simulink model "subsystem_118_bus"  (R2025b)
settings: Solver=ode45  StartTime=0.0  StopTime=Tstop  FixedStep=Ts  RelTol=1e-12  AbsTol=1e-12
values from neighbouring files (symbols this model uses):
  Imax = 15    [config_file.m]
  nominalInter =     [nominalInter.mat]
  nominalU =     [nominalU.mat]
  nominalY =     [nominalY.mat]
  sub = struct    [main_sub_118_bus.m]
  sys_j = sys_j(1:end-1)    [IBR_modelGenerator.m]
  sys_j_AA = sys_j    [modularMOR_main.m]
  sys_j_BT = sys_j    [modularMOR_main.m]
  Tstep_gfl = 0.1    [main_sub_118_bus.m]
  Tstep_gfm = 0.1    [main_sub_118_bus.m]
  w = 2*pi*50    (= 314.159265359)    [config_file.m]    (also in mirrorMimoWeightedFrequencyData.m = w(:); modularMOR_main.m = w(:).'; plotTest.m = w(:).')
undefined symbols (not defined in the file or in its folder): con_sub, linSys1, linSys2, linSys3
libraries: simulink x10
(part 6 of 6)

== system subsystem_118_bus/Subsystem3/area3/ibr/gfl/pll_pi ==
  "  " : Inport
  Integrator : Integrator  ContinuousStateAttributes='gfl_pll'
  Ki : Gain  Gain=Subsystem.gfl_gains.kipll
  Kp : Gain  Gain=Subsystem.gfl_gains.kppll
  Sum : Sum  Inputs=|++
  " " : Outport
  wires:
  Kp/1 -> Sum/1
  Integrator/1 -> Sum/2
  Ki/1 -> Integrator/1
  "  "/1 -> Ki/1, Kp/1
  Sum/1 -> " "/1

== system subsystem_118_bus/Subsystem3/area3/ibr/gfl/simplified current loop d-axis ==
  " " : Inport
  Gain : Gain  Gain=Subsystem.gfl.i_loop_w
  Integrator1 : Integrator  InitialCondition=Subsystem.gfl.i_d  ContinuousStateAttributes='gfl_id_ctrl'
  Sum2 : Sum  Inputs=-+
  "  " : Outport
  wires:
  Gain/1 -> Integrator1/1
  Integrator1/1 -> "  "/1, Sum2/1
  Sum2/1 -> Gain/1
  " "/1 -> Sum2/2

== system subsystem_118_bus/Subsystem3/area3/ibr/gfl/simplified current loop q-axis ==
  i_gfl_q : Inport
  Gain : Gain  Gain=Subsystem.gfl.i_loop_w
  Integrator1 : Integrator  InitialCondition=Subsystem.gfl.i_q  ContinuousStateAttributes='gfl_iq_ctrl'
  Sum2 : Sum  Inputs=-+
  igfl_q : Outport
  wires:
  Gain/1 -> Integrator1/1
  Integrator1/1 -> igfl_q/1, Sum2/1
  Sum2/1 -> Gain/1
  i_gfl_q/1 -> Sum2/2

== system subsystem_118_bus/Subsystem3/area3/ibr/gfl/v measurement delay ==
  in : Inport
  Integrator1 : Integrator  InitialCondition=Subsystem.gfl.v_ref  ContinuousStateAttributes='gfl_v_m'
  Sum2 : Sum  Inputs=-+
  v_meas_bw : Gain  Gain=Subsystem.gfl.v_meas_w
  out : Outport
  wires:
  in/1 -> Sum2/2
  Sum2/1 -> v_meas_bw/1
  Integrator1/1 -> Sum2/1, out/1
  v_meas_bw/1 -> Integrator1/1

== system subsystem_118_bus/Subsystem3/area3/ibr/gfl/v_loop_pi ==
  "  " : Inport
  Integrator : Integrator  ContinuousStateAttributes='gfl_v_ctrl'
  Ki : Gain  Gain=Subsystem.gfl_gains.kiv
  Kp : Gain  Gain=Subsystem.gfl_gains.kpv
  Sum : Sum  Inputs=|++
  " " : Outport
  wires:
  Kp/1 -> Sum/1
  Integrator/1 -> Sum/2
  Ki/1 -> Integrator/1
  "  "/1 -> Ki/1, Kp/1
  Sum/1 -> " "/1

== system subsystem_118_bus/Subsystem3/area3/ibr/gfm/DQ//dq ==
  D_quantity : Inport
  Q_quantity : Inport  Port=2
  theta : Inport  Port=3
  Complex to Magnitude-Angle : ComplexToMagnitudeAngle
  Complex to Real-Imag : ComplexToRealImag
  Magnitude-Angle to Complex : MagnitudeAngleToComplex
  Real-Imag to Complex : RealImagToComplex
  Sum : Sum  Inputs=|+-
  d_quantity : Outport
  q_quantity : Outport  Port=2
  wires:
  D_quantity/1 -> Real-Imag to Complex/1
  Complex to Magnitude-Angle/2 -> Sum/1
  Complex to Magnitude-Angle/1 -> Magnitude-Angle to Complex/1
  Real-Imag to Complex/1 -> Complex to Magnitude-Angle/1
  Sum/1 -> Magnitude-Angle to Complex/2
  Q_quantity/1 -> Real-Imag to Complex/2
  Magnitude-Angle to Complex/1 -> Complex to Real-Imag/1
  Complex to Real-Imag/1 -> d_quantity/1
  Complex to Real-Imag/2 -> q_quantity/1
  theta/1 -> Sum/2

== system subsystem_118_bus/Subsystem3/area3/ibr/gfm/Subsystem1 ==
  vbDQ : Inport
  IbDQ : Inport  Port=2
  Complex to Real-Imag : ComplexToRealImag
  Complex to Real-Imag1 : ComplexToRealImag
  Product{,1..3} (4 alike) : Product
  Sum : Sum
  Sum1 : Sum  Inputs=+-
  Pm : Outport
  Qm : Outport  Port=2
  wires:
  Product/1 -> Sum/1
  Product1/1 -> Sum/2
  Sum/1 -> Pm/1
  Sum1/1 -> Qm/1
  Product3/1 -> Sum1/2
  Product2/1 -> Sum1/1
  [vbQ] -> Product2/1
  [IbD] -> Product2/2
  [vbD] -> Product3/1
  [IbQ] -> Product3/2
  [vbD] -> Product/1
  [IbD] -> Product/2
  [IbQ] -> Product1/2
  [vbQ] -> Product1/1
  vbDQ/1 -> Complex to Real-Imag/1
  Complex to Real-Imag/1 -> [vbD]
  Complex to Real-Imag/2 -> [vbQ]
  IbDQ/1 -> Complex to Real-Imag1/1
  Complex to Real-Imag1/1 -> [IbD]
  Complex to Real-Imag1/2 -> [IbQ]

== system subsystem_118_bus/Subsystem3/area3/ibr/gfm/dq//DQ ==
  d-quantity : Inport
  q-quantity : Inport  Port=2
  theta : Inport  Port=3
  Complex to Magnitude-Angle : ComplexToMagnitudeAngle
  Complex to Real-Imag : ComplexToRealImag
  Magnitude-Angle to Complex : MagnitudeAngleToComplex
  Real-Imag to Complex : RealImagToComplex
  Sum : Sum  Inputs=|++
  D-quantity : Outport
  Q-quantity : Outport  Port=2
  wires:
  d-quantity/1 -> Real-Imag to Complex/1
  Complex to Magnitude-Angle/2 -> Sum/1
  Complex to Magnitude-Angle/1 -> Magnitude-Angle to Complex/1
  Real-Imag to Complex/1 -> Complex to Magnitude-Angle/1
  Sum/1 -> Magnitude-Angle to Complex/2
  q-quantity/1 -> Real-Imag to Complex/2
  Magnitude-Angle to Complex/1 -> Complex to Real-Imag/1
  Complex to Real-Imag/1 -> D-quantity/1
  Complex to Real-Imag/2 -> Q-quantity/1
  theta/1 -> Sum/2

== system subsystem_118_bus/Subsystem3/area3/ibr/gfm/filter capacitor dynamics ==
  i_cf_d : Inport
  w : Inport  Port=2
  i_cf_q : Inport  Port=3
  1/C_gfm : Gain  Gain=1./Subsystem.gfm.c
  "1/C_gfm " : Gain  Gain=1./Subsystem.gfm.c
  Display : Display
  Integrator : Integrator  InitialCondition=Subsystem.gfm.v_d  ContinuousStateAttributes='gfm_vd'
  Integrator1 : Integrator  InitialCondition=Subsystem.gfm.v_q  ContinuousStateAttributes='gfm_vq'
  Product : Product
  Product1 : Product
  Sum2 : Sum  Inputs=+-
  Sum3 : Sum
  v_gfl_d : Outport
  v_gfl_q : Outport  Port=2
  wires:
  w/1 -> [ws]
  [ws] -> Product/1
  Integrator/1 -> Product1/1, v_gfl_d/1
  Integrator1/1 -> Product/2, v_gfl_q/1
  [ws] -> Product1/2
  Sum3/1 -> Display/1, Integrator/1
  Sum2/1 -> Integrator1/1
  1/C_gfm/1 -> Sum3/2
  Product/1 -> Sum3/1
  "1/C_gfm "/1 -> Sum2/1
  Product1/1 -> Sum2/2
  i_cf_d/1 -> 1/C_gfm/1
  i_cf_q/1 -> "1/C_gfm "/1

== system subsystem_118_bus/Subsystem3/area3/ibr/gfm/p measurement delay ==
  in : Inport
  Integrator1 : Integrator  InitialCondition=Subsystem.gfm.p_ref  ContinuousStateAttributes='gfm_p_m'
  Sum2 : Sum  Inputs=-+
  p_meas_bw : Gain  Gain=Subsystem.gfm.p_meas_w
  out : Outport
  wires:
  in/1 -> Sum2/2
  Sum2/1 -> p_meas_bw/1
  Integrator1/1 -> Sum2/1, out/1
  p_meas_bw/1 -> Integrator1/1

== system subsystem_118_bus/Subsystem3/area3/ibr/gfm/q measurement delay ==
  in : Inport
  Integrator1 : Integrator  InitialCondition=Subsystem.gfm.q_ref  ContinuousStateAttributes='gfm_q_m'
  Sum2 : Sum  Inputs=-+
  p_meas_bw : Gain  Gain=Subsystem.gfm.p_meas_w
  out : Outport
  wires:
  p_meas_bw/1 -> Integrator1/1
  Integrator1/1 -> out/1, Sum2/1
  Sum2/1 -> p_meas_bw/1
  in/1 -> Sum2/2

== system subsystem_118_bus/Subsystem3/area3/ibr/gfm/simplified current loop d-axis ==
  " " : Inport
  Display : Display
  Gain : Gain  Gain=Subsystem.gfm.i_loop_w
  Integrator1 : Integrator  InitialCondition=Subsystem.gfm.i_d  ContinuousStateAttributes='gfm_id_ctrl'
  Sum2 : Sum  Inputs=-+
  "  " : Outport
  wires:
  Gain/1 -> Display/1, Integrator1/1
  Integrator1/1 -> "  "/1, Sum2/1
  Sum2/1 -> Gain/1
  " "/1 -> Sum2/2

== system subsystem_118_bus/Subsystem3/area3/ibr/gfm/simplified current loop q-axis ==
  " " : Inport
  Gain : Gain  Gain=Subsystem.gfm.i_loop_w
  Integrator1 : Integrator  InitialCondition=Subsystem.gfm.i_q  ContinuousStateAttributes='gfm_iq_ctrl'
  Sum2 : Sum  Inputs=-+
  "  " : Outport
  wires:
  " "/1 -> Sum2/2
  Sum2/1 -> Gain/1
  Integrator1/1 -> Sum2/1, "  "/1
  Gain/1 -> Integrator1/1

== system subsystem_118_bus/Subsystem3/area3/ibr/gfm/v measurement delay ==
  in : Inport
  Integrator1 : Integrator  InitialCondition=Subsystem.gfm.v_ref  ContinuousStateAttributes='gfm_v_m'
  Sum2 : Sum  Inputs=-+
  v_meas_bw : Gain  Gain=Subsystem.gfm.q_meas_w
  out : Outport
  wires:
  v_meas_bw/1 -> Integrator1/1
  Integrator1/1 -> out/1, Sum2/1
  Sum2/1 -> v_meas_bw/1
  in/1 -> Sum2/2

== system subsystem_118_bus/Subsystem3/area3/ibr/gfm/vd_loop_pi ==
  "  " : Inport
  Integrator : Integrator  ContinuousStateAttributes='gfm_vd_ctrl'
  Ki : Gain  Gain=Subsystem.gfm_gains.vd_ki
  Kp : Gain  Gain=Subsystem.gfm_gains.vd_kp
  Sum : Sum  Inputs=|++
  " " : Outport
  wires:
  Kp/1 -> Sum/1
  Integrator/1 -> Sum/2
  Ki/1 -> Integrator/1
  "  "/1 -> Ki/1, Kp/1
  Sum/1 -> " "/1

== system subsystem_118_bus/Subsystem3/area3/ibr/gfm/vq_loop_pi ==
  "  " : Inport
  Integrator : Integrator  ContinuousStateAttributes='gfm_vq_ctrl'
  Ki : Gain  Gain=Subsystem.gfm_gains.vq_ki
  Kp : Gain  Gain=Subsystem.gfm_gains.vq_kp
  Sum : Sum  Inputs=|++
  " " : Outport
  wires:
  Sum/1 -> " "/1
  "  "/1 -> Kp/1, Ki/1
  Ki/1 -> Integrator/1
  Integrator/1 -> Sum/2
  Kp/1 -> Sum/1

== system subsystem_118_bus/Subsystem3/area3/non_ibr/floating buses/line charging dynamics ==
  note: I am multiplying here by negative
  note: I am multiplying here by negative
  i_float_D : Inport
  i_float_Q : Inport  Port=2
  " " : Integrator  InitialCondition=Subsystem.float.v_D  ContinuousStateAttributes='floatvD'
  1/C_float : Gain  Gain=-1./Subsystem.float.c
  "1/C_float " : Gain  Gain=-1./Subsystem.float.c
  Constant : Constant  Value=w
  Integrator1 : Integrator  InitialCondition=Subsystem.float.v_Q  ContinuousStateAttributes='floatvQ'
  Product : Product
  Product1 : Product
  Sum2 : Sum  Inputs=+-
  Sum3 : Sum
  v_float_D : Outport
  v_float_Q : Outport  Port=2
  wires:
  " "/1 -> Product1/1, v_float_D/1
  Integrator1/1 -> v_float_Q/1, Product/2
  [ws] -> Product1/2
  Sum3/1 -> " "/1
  Sum2/1 -> Integrator1/1
  1/C_float/1 -> Sum3/2
  Product/1 -> Sum3/1
  "1/C_float "/1 -> Sum2/1
  Product1/1 -> Sum2/2
  i_float_D/1 -> 1/C_float/1
  i_float_Q/1 -> "1/C_float "/1
  [ws] -> Product/1
  Constant/1 -> [ws]

== system subsystem_118_bus/Subsystem3/area3/non_ibr/load buses/Subsystem ==
  p : Inport
  q : Inport  Port=2
  vD : Inport  Port=3
  vQ : Inport  Port=4
  Complex to Real-Imag : ComplexToRealImag
  Conj : Math  Operator=conj
  Divide : Product  Inputs=*/
  Real-Imag to Complex : RealImagToComplex
  Real-Imag to Complex1 : RealImagToComplex
  i_inj_load_d : Outport
  i_inj_load_q : Outport  Port=2
  wires:
  q/1 -> Real-Imag to Complex/2
  Real-Imag to Complex1/1 -> Divide/2
  Divide/1 -> Conj/1
  Complex to Real-Imag/2 -> i_inj_load_q/1
  Real-Imag to Complex/1 -> Divide/1
  vQ/1 -> Real-Imag to Complex1/2
  vD/1 -> Real-Imag to Complex1/1
  Complex to Real-Imag/1 -> i_inj_load_d/1
  p/1 -> Real-Imag to Complex/1
  Conj/1 -> Complex to Real-Imag/1

== system subsystem_118_bus/Subsystem3/area3/non_ibr/load buses/line charging dynamics ==
  i_load_c_D : Inport
  i_load_c_Q : Inport  Port=2
  " " : Integrator  InitialCondition=Subsystem.load1.v_D  ContinuousStateAttributes='loadvD'
  1/C_load : Gain  Gain=1./Subsystem.load1.c
  "1/C_load " : Gain  Gain=1./Subsystem.load1.c
  Constant : Constant  Value=w
  Integrator1 : Integrator  InitialCondition=Subsystem.load1.v_Q  ContinuousStateAttributes='loadvQ'
  Product : Product
  Product1 : Product
  Sum2 : Sum  Inputs=+-
  Sum3 : Sum
  v_load_D : Outport
  v_load_Q : Outport  Port=2
  wires:
  [ws] -> Product/1
  " "/1 -> Product1/1, v_load_D/1
  Integrator1/1 -> v_load_Q/1, Product/2
  [ws] -> Product1/2
  Sum3/1 -> " "/1
  Sum2/1 -> Integrator1/1
  1/C_load/1 -> Sum3/2
  Product/1 -> Sum3/1
  "1/C_load "/1 -> Sum2/1
  Product1/1 -> Sum2/2
  i_load_c_D/1 -> 1/C_load/1
  i_load_c_Q/1 -> "1/C_load "/1
  Constant/1 -> [ws]

== system subsystem_118_bus/Linear 118 Bus FOM/Subsystem3/area3/ibr/gfl/DQ//dq ==
  D_quantity : Inport
  Q_quantity : Inport  Port=2
  theta : Inport  Port=3
  Complex to Magnitude-Angle : ComplexToMagnitudeAngle
  Complex to Real-Imag : ComplexToRealImag
  Magnitude-Angle to Complex : MagnitudeAngleToComplex
  Real-Imag to Complex : RealImagToComplex
  Sum : Sum  Inputs=|+-
  d_quantity : Outport
  q_quantity : Outport  Port=2
  wires:
  D_quantity/1 -> Real-Imag to Complex/1
  Complex to Magnitude-Angle/2 -> Sum/1
  Complex to Magnitude-Angle/1 -> Magnitude-Angle to Complex/1
  Real-Imag to Complex/1 -> Complex to Magnitude-Angle/1
  Sum/1 -> Magnitude-Angle to Complex/2
  Q_quantity/1 -> Real-Imag to Complex/2
  Magnitude-Angle to Complex/1 -> Complex to Real-Imag/1
  Complex to Real-Imag/1 -> d_quantity/1
  Complex to Real-Imag/2 -> q_quantity/1
  theta/1 -> Sum/2

== system subsystem_118_bus/Linear 118 Bus FOM/Subsystem3/area3/ibr/gfl/Subsystem ==
  vbDQ : Inport
  Abs : Abs  SaturateOnIntegerOverflow=off
  Vm : Outport
  wires:
  Abs/1 -> Vm/1
  vbDQ/1 -> Abs/1

== system subsystem_118_bus/Linear 118 Bus FOM/Subsystem3/area3/ibr/gfl/Subsystem1 ==
  vbDQ : Inport
  IbDQ : Inport  Port=2
  Complex to Real-Imag : ComplexToRealImag
  Complex to Real-Imag1 : ComplexToRealImag
  Product{,1..3} (4 alike) : Product
  Sum : Sum
  Sum1 : Sum  Inputs=+-
  Pm : Outport
  Qm : Outport  Port=2
  wires:
  Product/1 -> Sum/1
  Product1/1 -> Sum/2
  Sum/1 -> Pm/1
  Sum1/1 -> Qm/1
  Product3/1 -> Sum1/2
  Product2/1 -> Sum1/1
  [vbQ] -> Product2/1
  [IbD] -> Product2/2
  [vbD] -> Product3/1
  [IbQ] -> Product3/2
  [vbD] -> Product/1
  [IbD] -> Product/2
  [IbQ] -> Product1/2
  [vbQ] -> Product1/1
  vbDQ/1 -> Complex to Real-Imag/1
  Complex to Real-Imag/1 -> [vbD]
  Complex to Real-Imag/2 -> [vbQ]
  IbDQ/1 -> Complex to Real-Imag1/1
  Complex to Real-Imag1/1 -> [IbD]
  Complex to Real-Imag1/2 -> [IbQ]

== system subsystem_118_bus/Linear 118 Bus FOM/Subsystem3/area3/ibr/gfl/dq//DQ ==
  d-quantity : Inport
  q-quantity : Inport  Port=2
  theta : Inport  Port=3
  Complex to Magnitude-Angle : ComplexToMagnitudeAngle
  Complex to Real-Imag : ComplexToRealImag
  Magnitude-Angle to Complex : MagnitudeAngleToComplex
  Real-Imag to Complex : RealImagToComplex
  Sum : Sum  Inputs=|++
  D-quantity : Outport
  Q-quantity : Outport  Port=2
  wires:
  d-quantity/1 -> Real-Imag to Complex/1
  Complex to Magnitude-Angle/2 -> Sum/1
  Complex to Magnitude-Angle/1 -> Magnitude-Angle to Complex/1
  Real-Imag to Complex/1 -> Complex to Magnitude-Angle/1
  Sum/1 -> Magnitude-Angle to Complex/2
  q-quantity/1 -> Real-Imag to Complex/2
  Magnitude-Angle to Complex/1 -> Complex to Real-Imag/1
  Complex to Real-Imag/1 -> D-quantity/1
  Complex to Real-Imag/2 -> Q-quantity/1
  theta/1 -> Sum/2

== system subsystem_118_bus/Linear 118 Bus FOM/Subsystem3/area3/ibr/gfl/filter capacitor dynamics ==
  i_cf_d : Inport
  w : Inport  Port=2
  i_cf_q : Inport  Port=3
  1/C_gfl_pv : Gain  Gain=1./Subsystem.gfl.c
  "1/C_gfl_pv " : Gain  Gain=1./Subsystem.gfl.c
  Integrator : Integrator  InitialCondition=Subsystem.gfl.v_d  ContinuousStateAttributes='gfl_vd'
  Integrator1 : Integrator  InitialCondition=Subsystem.gfl.v_q  ContinuousStateAttributes='gfl_vq'
  Product : Product
  Product1 : Product
  Sum2 : Sum  Inputs=+-
  Sum3 : Sum
  v_gfl_d : Outport
  v_gfl_q : Outport  Port=2
  wires:
  w/1 -> [ws]
  [ws] -> Product/1
  Integrator/1 -> Product1/1, v_gfl_d/1
  Integrator1/1 -> Product/2, v_gfl_q/1
  [ws] -> Product1/2
  Sum3/1 -> Integrator/1
  Sum2/1 -> Integrator1/1
  1/C_gfl_pv/1 -> Sum3/2
  Product/1 -> Sum3/1
  "1/C_gfl_pv "/1 -> Sum2/1
  Product1/1 -> Sum2/2
  i_cf_d/1 -> 1/C_gfl_pv/1
  i_cf_q/1 -> "1/C_gfl_pv "/1

== system subsystem_118_bus/Linear 118 Bus FOM/Subsystem3/area3/ibr/gfl/p measurement delay ==
  in : Inport
  Integrator1 : Integrator  InitialCondition=Subsystem.gfl.p_ref  ContinuousStateAttributes='gfl_p_m'
  Sum2 : Sum  Inputs=-+
  p_meas_bw : Gain  Gain=Subsystem.gfl.p_meas_w
  out : Outport
  wires:
  in/1 -> Sum2/2
  Sum2/1 -> p_meas_bw/1
  Integrator1/1 -> Sum2/1, out/1
  p_meas_bw/1 -> Integrator1/1

== system subsystem_118_bus/Linear 118 Bus FOM/Subsystem3/area3/ibr/gfl/p_loop_pi ==
  "  " : Inport
  Integrator : Integrator  ContinuousStateAttributes='gfl_p_ctrl'
  Ki : Gain  Gain=Subsystem.gfl_gains.kip
  Kp : Gain  Gain=Subsystem.gfl_gains.kpp
  Sum : Sum  Inputs=|++
  " " : Outport
  wires:
  Kp/1 -> Sum/1
  Integrator/1 -> Sum/2
  Ki/1 -> Integrator/1
  "  "/1 -> Ki/1, Kp/1
  Sum/1 -> " "/1

== system subsystem_118_bus/Linear 118 Bus FOM/Subsystem3/area3/ibr/gfl/pll_lpf ==
  LPF_input : Inport
  Integrator1 : Integrator  ContinuousStateAttributes='gfl_pll_lpf'
  Sum2 : Sum  Inputs=-+
  pll_lpf_bw : Gain  Gain=Subsystem.gfl.pll_lpf_w
  LPF_output : Outport
  wires:
  pll_lpf_bw/1 -> Integrator1/1
  Integrator1/1 -> LPF_output/1, Sum2/1
  Sum2/1 -> pll_lpf_bw/1
  LPF_input/1 -> Sum2/2

== system subsystem_118_bus/Linear 118 Bus FOM/Subsystem3/area3/ibr/gfl/pll_pi ==
  "  " : Inport
  Integrator : Integrator  ContinuousStateAttributes='gfl_pll'
  Ki : Gain  Gain=Subsystem.gfl_gains.kipll
  Kp : Gain  Gain=Subsystem.gfl_gains.kppll
  Sum : Sum  Inputs=|++
  " " : Outport
  wires:
  Kp/1 -> Sum/1
  Integrator/1 -> Sum/2
  Ki/1 -> Integrator/1
  "  "/1 -> Ki/1, Kp/1
  Sum/1 -> " "/1

== system subsystem_118_bus/Linear 118 Bus FOM/Subsystem3/area3/ibr/gfl/simplified current loop d-axis ==
  " " : Inport
  Gain : Gain  Gain=Subsystem.gfl.i_loop_w
  Integrator1 : Integrator  InitialCondition=Subsystem.gfl.i_d  ContinuousStateAttributes='gfl_id_ctrl'
  Sum2 : Sum  Inputs=-+
  "  " : Outport
  wires:
  Gain/1 -> Integrator1/1
  Integrator1/1 -> "  "/1, Sum2/1
  Sum2/1 -> Gain/1
  " "/1 -> Sum2/2

== system subsystem_118_bus/Linear 118 Bus FOM/Subsystem3/area3/ibr/gfl/simplified current loop q-axis ==
  i_gfl_q : Inport
  Gain : Gain  Gain=Subsystem.gfl.i_loop_w
  Integrator1 : Integrator  InitialCondition=Subsystem.gfl.i_q  ContinuousStateAttributes='gfl_iq_ctrl'
  Sum2 : Sum  Inputs=-+
  igfl_q : Outport
  wires:
  Gain/1 -> Integrator1/1
  Integrator1/1 -> igfl_q/1, Sum2/1
  Sum2/1 -> Gain/1
  i_gfl_q/1 -> Sum2/2

== system subsystem_118_bus/Linear 118 Bus FOM/Subsystem3/area3/ibr/gfl/v measurement delay ==
  in : Inport
  Integrator1 : Integrator  InitialCondition=Subsystem.gfl.v_ref  ContinuousStateAttributes='gfl_v_m'
  Sum2 : Sum  Inputs=-+
  v_meas_bw : Gain  Gain=Subsystem.gfl.v_meas_w
  out : Outport
  wires:
  in/1 -> Sum2/2
  Sum2/1 -> v_meas_bw/1
  Integrator1/1 -> Sum2/1, out/1
  v_meas_bw/1 -> Integrator1/1

== system subsystem_118_bus/Linear 118 Bus FOM/Subsystem3/area3/ibr/gfl/v_loop_pi ==
  "  " : Inport
  Integrator : Integrator  ContinuousStateAttributes='gfl_v_ctrl'
  Ki : Gain  Gain=Subsystem.gfl_gains.kiv
  Kp : Gain  Gain=Subsystem.gfl_gains.kpv
  Sum : Sum  Inputs=|++
  " " : Outport
  wires:
  Kp/1 -> Sum/1
  Integrator/1 -> Sum/2
  Ki/1 -> Integrator/1
  "  "/1 -> Ki/1, Kp/1
  Sum/1 -> " "/1

== system subsystem_118_bus/Linear 118 Bus FOM/Subsystem3/area3/ibr/gfm/DQ//dq ==
  D_quantity : Inport
  Q_quantity : Inport  Port=2
  theta : Inport  Port=3
  Complex to Magnitude-Angle : ComplexToMagnitudeAngle
  Complex to Real-Imag : ComplexToRealImag
  Magnitude-Angle to Complex : MagnitudeAngleToComplex
  Real-Imag to Complex : RealImagToComplex
  Sum : Sum  Inputs=|+-
  d_quantity : Outport
  q_quantity : Outport  Port=2
  wires:
  D_quantity/1 -> Real-Imag to Complex/1
  Complex to Magnitude-Angle/2 -> Sum/1
  Complex to Magnitude-Angle/1 -> Magnitude-Angle to Complex/1
  Real-Imag to Complex/1 -> Complex to Magnitude-Angle/1
  Sum/1 -> Magnitude-Angle to Complex/2
  Q_quantity/1 -> Real-Imag to Complex/2
  Magnitude-Angle to Complex/1 -> Complex to Real-Imag/1
  Complex to Real-Imag/1 -> d_quantity/1
  Complex to Real-Imag/2 -> q_quantity/1
  theta/1 -> Sum/2

== system subsystem_118_bus/Linear 118 Bus FOM/Subsystem3/area3/ibr/gfm/Subsystem1 ==
  vbDQ : Inport
  IbDQ : Inport  Port=2
  Complex to Real-Imag : ComplexToRealImag
  Complex to Real-Imag1 : ComplexToRealImag
  Product{,1..3} (4 alike) : Product
  Sum : Sum
  Sum1 : Sum  Inputs=+-
  Pm : Outport
  Qm : Outport  Port=2
  wires:
  Product/1 -> Sum/1
  Product1/1 -> Sum/2
  Sum/1 -> Pm/1
  Sum1/1 -> Qm/1
  Product3/1 -> Sum1/2
  Product2/1 -> Sum1/1
  [vbQ] -> Product2/1
  [IbD] -> Product2/2
  [vbD] -> Product3/1
  [IbQ] -> Product3/2
  [vbD] -> Product/1
  [IbD] -> Product/2
  [IbQ] -> Product1/2
  [vbQ] -> Product1/1
  vbDQ/1 -> Complex to Real-Imag/1
  Complex to Real-Imag/1 -> [vbD]
  Complex to Real-Imag/2 -> [vbQ]
  IbDQ/1 -> Complex to Real-Imag1/1
  Complex to Real-Imag1/1 -> [IbD]
  Complex to Real-Imag1/2 -> [IbQ]

== system subsystem_118_bus/Linear 118 Bus FOM/Subsystem3/area3/ibr/gfm/dq//DQ ==
  d-quantity : Inport
  q-quantity : Inport  Port=2
  theta : Inport  Port=3
  Complex to Magnitude-Angle : ComplexToMagnitudeAngle
  Complex to Real-Imag : ComplexToRealImag
  Magnitude-Angle to Complex : MagnitudeAngleToComplex
  Real-Imag to Complex : RealImagToComplex
  Sum : Sum  Inputs=|++
  D-quantity : Outport
  Q-quantity : Outport  Port=2
  wires:
  d-quantity/1 -> Real-Imag to Complex/1
  Complex to Magnitude-Angle/2 -> Sum/1
  Complex to Magnitude-Angle/1 -> Magnitude-Angle to Complex/1
  Real-Imag to Complex/1 -> Complex to Magnitude-Angle/1
  Sum/1 -> Magnitude-Angle to Complex/2
  q-quantity/1 -> Real-Imag to Complex/2
  Magnitude-Angle to Complex/1 -> Complex to Real-Imag/1
  Complex to Real-Imag/1 -> D-quantity/1
  Complex to Real-Imag/2 -> Q-quantity/1
  theta/1 -> Sum/2

== system subsystem_118_bus/Linear 118 Bus FOM/Subsystem3/area3/ibr/gfm/filter capacitor dynamics ==
  i_cf_d : Inport
  w : Inport  Port=2
  i_cf_q : Inport  Port=3
  1/C_gfm : Gain  Gain=1./Subsystem.gfm.c
  "1/C_gfm " : Gain  Gain=1./Subsystem.gfm.c
  Display : Display
  Integrator : Integrator  InitialCondition=Subsystem.gfm.v_d  ContinuousStateAttributes='gfm_vd'
  Integrator1 : Integrator  InitialCondition=Subsystem.gfm.v_q  ContinuousStateAttributes='gfm_vq'
  Product : Product
  Product1 : Product
  Sum2 : Sum  Inputs=+-
  Sum3 : Sum
  v_gfl_d : Outport
  v_gfl_q : Outport  Port=2
  wires:
  w/1 -> [ws]
  [ws] -> Product/1
  Integrator/1 -> Product1/1, v_gfl_d/1
  Integrator1/1 -> Product/2, v_gfl_q/1
  [ws] -> Product1/2
  Sum3/1 -> Display/1, Integrator/1
  Sum2/1 -> Integrator1/1
  1/C_gfm/1 -> Sum3/2
  Product/1 -> Sum3/1
  "1/C_gfm "/1 -> Sum2/1
  Product1/1 -> Sum2/2
  i_cf_d/1 -> 1/C_gfm/1
  i_cf_q/1 -> "1/C_gfm "/1

== system subsystem_118_bus/Linear 118 Bus FOM/Subsystem3/area3/ibr/gfm/p measurement delay ==
  in : Inport
  Integrator1 : Integrator  InitialCondition=Subsystem.gfm.p_ref  ContinuousStateAttributes='gfm_p_m'
  Sum2 : Sum  Inputs=-+
  p_meas_bw : Gain  Gain=Subsystem.gfm.p_meas_w
  out : Outport
  wires:
  in/1 -> Sum2/2
  Sum2/1 -> p_meas_bw/1
  Integrator1/1 -> Sum2/1, out/1
  p_meas_bw/1 -> Integrator1/1

== system subsystem_118_bus/Linear 118 Bus FOM/Subsystem3/area3/ibr/gfm/q measurement delay ==
  in : Inport
  Integrator1 : Integrator  InitialCondition=Subsystem.gfm.q_ref  ContinuousStateAttributes='gfm_q_m'
  Sum2 : Sum  Inputs=-+
  p_meas_bw : Gain  Gain=Subsystem.gfm.p_meas_w
  out : Outport
  wires:
  p_meas_bw/1 -> Integrator1/1
  Integrator1/1 -> out/1, Sum2/1
  Sum2/1 -> p_meas_bw/1
  in/1 -> Sum2/2

== system subsystem_118_bus/Linear 118 Bus FOM/Subsystem3/area3/ibr/gfm/simplified current loop d-axis ==
  " " : Inport
  Display : Display
  Gain : Gain  Gain=Subsystem.gfm.i_loop_w
  Integrator1 : Integrator  InitialCondition=Subsystem.gfm.i_d  ContinuousStateAttributes='gfm_id_ctrl'
  Sum2 : Sum  Inputs=-+
  "  " : Outport
  wires:
  Gain/1 -> Display/1, Integrator1/1
  Integrator1/1 -> "  "/1, Sum2/1
  Sum2/1 -> Gain/1
  " "/1 -> Sum2/2

== system subsystem_118_bus/Linear 118 Bus FOM/Subsystem3/area3/ibr/gfm/simplified current loop q-axis ==
  " " : Inport
  Gain : Gain  Gain=Subsystem.gfm.i_loop_w
  Integrator1 : Integrator  InitialCondition=Subsystem.gfm.i_q  ContinuousStateAttributes='gfm_iq_ctrl'
  Sum2 : Sum  Inputs=-+
  "  " : Outport
  wires:
  " "/1 -> Sum2/2
  Sum2/1 -> Gain/1
  Integrator1/1 -> Sum2/1, "  "/1
  Gain/1 -> Integrator1/1

== system subsystem_118_bus/Linear 118 Bus FOM/Subsystem3/area3/ibr/gfm/v measurement delay ==
  in : Inport
  Integrator1 : Integrator  InitialCondition=Subsystem.gfm.v_ref  ContinuousStateAttributes='gfm_v_m'
  Sum2 : Sum  Inputs=-+
  v_meas_bw : Gain  Gain=Subsystem.gfm.q_meas_w
  out : Outport
  wires:
  v_meas_bw/1 -> Integrator1/1
  Integrator1/1 -> out/1, Sum2/1
  Sum2/1 -> v_meas_bw/1
  in/1 -> Sum2/2

== system subsystem_118_bus/Linear 118 Bus FOM/Subsystem3/area3/ibr/gfm/vd_loop_pi ==
  "  " : Inport
  Integrator : Integrator  ContinuousStateAttributes='gfm_vd_ctrl'
  Ki : Gain  Gain=Subsystem.gfm_gains.vd_ki
  Kp : Gain  Gain=Subsystem.gfm_gains.vd_kp
  Sum : Sum  Inputs=|++
  " " : Outport
  wires:
  Kp/1 -> Sum/1
  Integrator/1 -> Sum/2
  Ki/1 -> Integrator/1
  "  "/1 -> Ki/1, Kp/1
  Sum/1 -> " "/1

== system subsystem_118_bus/Linear 118 Bus FOM/Subsystem3/area3/ibr/gfm/vq_loop_pi ==
  "  " : Inport
  Integrator : Integrator  ContinuousStateAttributes='gfm_vq_ctrl'
  Ki : Gain  Gain=Subsystem.gfm_gains.vq_ki
  Kp : Gain  Gain=Subsystem.gfm_gains.vq_kp
  Sum : Sum  Inputs=|++
  " " : Outport
  wires:
  Sum/1 -> " "/1
  "  "/1 -> Kp/1, Ki/1
  Ki/1 -> Integrator/1
  Integrator/1 -> Sum/2
  Kp/1 -> Sum/1

== system subsystem_118_bus/Linear 118 Bus FOM/Subsystem3/area3/non_ibr/floating buses/line charging dynamics ==
  note: I am multiplying here by negative
  note: I am multiplying here by negative
  i_float_D : Inport
  i_float_Q : Inport  Port=2
  " " : Integrator  InitialCondition=Subsystem.float.v_D  ContinuousStateAttributes='floatvD'
  1/C_float : Gain  Gain=-1./Subsystem.float.c
  "1/C_float " : Gain  Gain=-1./Subsystem.float.c
  Constant : Constant  Value=w
  Integrator1 : Integrator  InitialCondition=Subsystem.float.v_Q  ContinuousStateAttributes='floatvQ'
  Product : Product
  Product1 : Product
  Sum2 : Sum  Inputs=+-
  Sum3 : Sum
  v_float_D : Outport
  v_float_Q : Outport  Port=2
  wires:
  " "/1 -> Product1/1, v_float_D/1
  Integrator1/1 -> v_float_Q/1, Product/2
  [ws] -> Product1/2
  Sum3/1 -> " "/1
  Sum2/1 -> Integrator1/1
  1/C_float/1 -> Sum3/2
  Product/1 -> Sum3/1
  "1/C_float "/1 -> Sum2/1
  Product1/1 -> Sum2/2
  i_float_D/1 -> 1/C_float/1
  i_float_Q/1 -> "1/C_float "/1
  [ws] -> Product/1
  Constant/1 -> [ws]

== system subsystem_118_bus/Linear 118 Bus FOM/Subsystem3/area3/non_ibr/load buses/Subsystem ==
  p : Inport
  q : Inport  Port=2
  vD : Inport  Port=3
  vQ : Inport  Port=4
  Complex to Real-Imag : ComplexToRealImag
  Conj : Math  Operator=conj
  Divide : Product  Inputs=*/
  Real-Imag to Complex : RealImagToComplex
  Real-Imag to Complex1 : RealImagToComplex
  i_inj_load_d : Outport
  i_inj_load_q : Outport  Port=2
  wires:
  q/1 -> Real-Imag to Complex/2
  Real-Imag to Complex1/1 -> Divide/2
  Divide/1 -> Conj/1
  Complex to Real-Imag/2 -> i_inj_load_q/1
  Real-Imag to Complex/1 -> Divide/1
  vQ/1 -> Real-Imag to Complex1/2
  vD/1 -> Real-Imag to Complex1/1
  Complex to Real-Imag/1 -> i_inj_load_d/1
  p/1 -> Real-Imag to Complex/1
  Conj/1 -> Complex to Real-Imag/1

== system subsystem_118_bus/Linear 118 Bus FOM/Subsystem3/area3/non_ibr/load buses/line charging dynamics ==
  i_load_c_D : Inport
  i_load_c_Q : Inport  Port=2
  " " : Integrator  InitialCondition=Subsystem.load1.v_D  ContinuousStateAttributes='loadvD'
  1/C_load : Gain  Gain=1./Subsystem.load1.c
  "1/C_load " : Gain  Gain=1./Subsystem.load1.c
  Constant : Constant  Value=w
  Integrator1 : Integrator  InitialCondition=Subsystem.load1.v_Q  ContinuousStateAttributes='loadvQ'
  Product : Product
  Product1 : Product
  Sum2 : Sum  Inputs=+-
  Sum3 : Sum
  v_load_D : Outport
  v_load_Q : Outport  Port=2
  wires:
  [ws] -> Product/1
  " "/1 -> Product1/1, v_load_D/1
  Integrator1/1 -> v_load_Q/1, Product/2
  [ws] -> Product1/2
  Sum3/1 -> " "/1
  Sum2/1 -> Integrator1/1
  1/C_load/1 -> Sum3/2
  Product/1 -> Sum3/1
  "1/C_load "/1 -> Sum2/1
  Product1/1 -> Sum2/2
  i_load_c_D/1 -> 1/C_load/1
  i_load_c_Q/1 -> "1/C_load "/1
  Constant/1 -> [ws]

== system subsystem_118_bus/Linear 118 Bus ROM/Subsystem3/area3/ibr/gfl/DQ//dq ==
  D_quantity : Inport
  Q_quantity : Inport  Port=2
  theta : Inport  Port=3
  Complex to Magnitude-Angle : ComplexToMagnitudeAngle
  Complex to Real-Imag : ComplexToRealImag
  Magnitude-Angle to Complex : MagnitudeAngleToComplex
  Real-Imag to Complex : RealImagToComplex
  Sum : Sum  Inputs=|+-
  d_quantity : Outport
  q_quantity : Outport  Port=2
  wires:
  D_quantity/1 -> Real-Imag to Complex/1
  Complex to Magnitude-Angle/2 -> Sum/1
  Complex to Magnitude-Angle/1 -> Magnitude-Angle to Complex/1
  Real-Imag to Complex/1 -> Complex to Magnitude-Angle/1
  Sum/1 -> Magnitude-Angle to Complex/2
  Q_quantity/1 -> Real-Imag to Complex/2
  Magnitude-Angle to Complex/1 -> Complex to Real-Imag/1
  Complex to Real-Imag/1 -> d_quantity/1
  Complex to Real-Imag/2 -> q_quantity/1
  theta/1 -> Sum/2

== system subsystem_118_bus/Linear 118 Bus ROM/Subsystem3/area3/ibr/gfl/Subsystem ==
  vbDQ : Inport
  Abs : Abs  SaturateOnIntegerOverflow=off
  Vm : Outport
  wires:
  Abs/1 -> Vm/1
  vbDQ/1 -> Abs/1

== system subsystem_118_bus/Linear 118 Bus ROM/Subsystem3/area3/ibr/gfl/Subsystem1 ==
  vbDQ : Inport
  IbDQ : Inport  Port=2
  Complex to Real-Imag : ComplexToRealImag
  Complex to Real-Imag1 : ComplexToRealImag
  Product{,1..3} (4 alike) : Product
  Sum : Sum
  Sum1 : Sum  Inputs=+-
  Pm : Outport
  Qm : Outport  Port=2
  wires:
  Product/1 -> Sum/1
  Product1/1 -> Sum/2
  Sum/1 -> Pm/1
  Sum1/1 -> Qm/1
  Product3/1 -> Sum1/2
  Product2/1 -> Sum1/1
  [vbQ] -> Product2/1
  [IbD] -> Product2/2
  [vbD] -> Product3/1
  [IbQ] -> Product3/2
  [vbD] -> Product/1
  [IbD] -> Product/2
  [IbQ] -> Product1/2
  [vbQ] -> Product1/1
  vbDQ/1 -> Complex to Real-Imag/1
  Complex to Real-Imag/1 -> [vbD]
  Complex to Real-Imag/2 -> [vbQ]
  IbDQ/1 -> Complex to Real-Imag1/1
  Complex to Real-Imag1/1 -> [IbD]
  Complex to Real-Imag1/2 -> [IbQ]

== system subsystem_118_bus/Linear 118 Bus ROM/Subsystem3/area3/ibr/gfl/dq//DQ ==
  d-quantity : Inport
  q-quantity : Inport  Port=2
  theta : Inport  Port=3
  Complex to Magnitude-Angle : ComplexToMagnitudeAngle
  Complex to Real-Imag : ComplexToRealImag
  Magnitude-Angle to Complex : MagnitudeAngleToComplex
  Real-Imag to Complex : RealImagToComplex
  Sum : Sum  Inputs=|++
  D-quantity : Outport
  Q-quantity : Outport  Port=2
  wires:
  d-quantity/1 -> Real-Imag to Complex/1
  Complex to Magnitude-Angle/2 -> Sum/1
  Complex to Magnitude-Angle/1 -> Magnitude-Angle to Complex/1
  Real-Imag to Complex/1 -> Complex to Magnitude-Angle/1
  Sum/1 -> Magnitude-Angle to Complex/2
  q-quantity/1 -> Real-Imag to Complex/2
  Magnitude-Angle to Complex/1 -> Complex to Real-Imag/1
  Complex to Real-Imag/1 -> D-quantity/1
  Complex to Real-Imag/2 -> Q-quantity/1
  theta/1 -> Sum/2

== system subsystem_118_bus/Linear 118 Bus ROM/Subsystem3/area3/ibr/gfl/filter capacitor dynamics ==
  i_cf_d : Inport
  w : Inport  Port=2
  i_cf_q : Inport  Port=3
  1/C_gfl_pv : Gain  Gain=1./Subsystem.gfl.c
  "1/C_gfl_pv " : Gain  Gain=1./Subsystem.gfl.c
  Integrator : Integrator  InitialCondition=Subsystem.gfl.v_d  ContinuousStateAttributes='gfl_vd'
  Integrator1 : Integrator  InitialCondition=Subsystem.gfl.v_q  ContinuousStateAttributes='gfl_vq'
  Product : Product
  Product1 : Product
  Sum2 : Sum  Inputs=+-
  Sum3 : Sum
  v_gfl_d : Outport
  v_gfl_q : Outport  Port=2
  wires:
  w/1 -> [ws]
  [ws] -> Product/1
  Integrator/1 -> Product1/1, v_gfl_d/1
  Integrator1/1 -> Product/2, v_gfl_q/1
  [ws] -> Product1/2
  Sum3/1 -> Integrator/1
  Sum2/1 -> Integrator1/1
  1/C_gfl_pv/1 -> Sum3/2
  Product/1 -> Sum3/1
  "1/C_gfl_pv "/1 -> Sum2/1
  Product1/1 -> Sum2/2
  i_cf_d/1 -> 1/C_gfl_pv/1
  i_cf_q/1 -> "1/C_gfl_pv "/1

== system subsystem_118_bus/Linear 118 Bus ROM/Subsystem3/area3/ibr/gfl/p measurement delay ==
  in : Inport
  Integrator1 : Integrator  InitialCondition=Subsystem.gfl.p_ref  ContinuousStateAttributes='gfl_p_m'
  Sum2 : Sum  Inputs=-+
  p_meas_bw : Gain  Gain=Subsystem.gfl.p_meas_w
  out : Outport
  wires:
  in/1 -> Sum2/2
  Sum2/1 -> p_meas_bw/1
  Integrator1/1 -> Sum2/1, out/1
  p_meas_bw/1 -> Integrator1/1

== system subsystem_118_bus/Linear 118 Bus ROM/Subsystem3/area3/ibr/gfl/p_loop_pi ==
  "  " : Inport
  Integrator : Integrator  ContinuousStateAttributes='gfl_p_ctrl'
  Ki : Gain  Gain=Subsystem.gfl_gains.kip
  Kp : Gain  Gain=Subsystem.gfl_gains.kpp
  Sum : Sum  Inputs=|++
  " " : Outport
  wires:
  Kp/1 -> Sum/1
  Integrator/1 -> Sum/2
  Ki/1 -> Integrator/1
  "  "/1 -> Ki/1, Kp/1
  Sum/1 -> " "/1

== system subsystem_118_bus/Linear 118 Bus ROM/Subsystem3/area3/ibr/gfl/pll_lpf ==
  LPF_input : Inport
  Integrator1 : Integrator  ContinuousStateAttributes='gfl_pll_lpf'
  Sum2 : Sum  Inputs=-+
  pll_lpf_bw : Gain  Gain=Subsystem.gfl.pll_lpf_w
  LPF_output : Outport
  wires:
  pll_lpf_bw/1 -> Integrator1/1
  Integrator1/1 -> LPF_output/1, Sum2/1
  Sum2/1 -> pll_lpf_bw/1
  LPF_input/1 -> Sum2/2

== system subsystem_118_bus/Linear 118 Bus ROM/Subsystem3/area3/ibr/gfl/pll_pi ==
  "  " : Inport
  Integrator : Integrator  ContinuousStateAttributes='gfl_pll'
  Ki : Gain  Gain=Subsystem.gfl_gains.kipll
  Kp : Gain  Gain=Subsystem.gfl_gains.kppll
  Sum : Sum  Inputs=|++
  " " : Outport
  wires:
  Kp/1 -> Sum/1
  Integrator/1 -> Sum/2
  Ki/1 -> Integrator/1
  "  "/1 -> Ki/1, Kp/1
  Sum/1 -> " "/1

== system subsystem_118_bus/Linear 118 Bus ROM/Subsystem3/area3/ibr/gfl/simplified current loop d-axis ==
  " " : Inport
  Gain : Gain  Gain=Subsystem.gfl.i_loop_w
  Integrator1 : Integrator  InitialCondition=Subsystem.gfl.i_d  ContinuousStateAttributes='gfl_id_ctrl'
  Sum2 : Sum  Inputs=-+
  "  " : Outport
  wires:
  Gain/1 -> Integrator1/1
  Integrator1/1 -> "  "/1, Sum2/1
  Sum2/1 -> Gain/1
  " "/1 -> Sum2/2

== system subsystem_118_bus/Linear 118 Bus ROM/Subsystem3/area3/ibr/gfl/simplified current loop q-axis ==
  i_gfl_q : Inport
  Gain : Gain  Gain=Subsystem.gfl.i_loop_w
  Integrator1 : Integrator  InitialCondition=Subsystem.gfl.i_q  ContinuousStateAttributes='gfl_iq_ctrl'
  Sum2 : Sum  Inputs=-+
  igfl_q : Outport
  wires:
  Gain/1 -> Integrator1/1
  Integrator1/1 -> igfl_q/1, Sum2/1
  Sum2/1 -> Gain/1
  i_gfl_q/1 -> Sum2/2

== system subsystem_118_bus/Linear 118 Bus ROM/Subsystem3/area3/ibr/gfl/v measurement delay ==
  in : Inport
  Integrator1 : Integrator  InitialCondition=Subsystem.gfl.v_ref  ContinuousStateAttributes='gfl_v_m'
  Sum2 : Sum  Inputs=-+
  v_meas_bw : Gain  Gain=Subsystem.gfl.v_meas_w
  out : Outport
  wires:
  in/1 -> Sum2/2
  Sum2/1 -> v_meas_bw/1
  Integrator1/1 -> Sum2/1, out/1
  v_meas_bw/1 -> Integrator1/1

== system subsystem_118_bus/Linear 118 Bus ROM/Subsystem3/area3/ibr/gfl/v_loop_pi ==
  "  " : Inport
  Integrator : Integrator  ContinuousStateAttributes='gfl_v_ctrl'
  Ki : Gain  Gain=Subsystem.gfl_gains.kiv
  Kp : Gain  Gain=Subsystem.gfl_gains.kpv
  Sum : Sum  Inputs=|++
  " " : Outport
  wires:
  Kp/1 -> Sum/1
  Integrator/1 -> Sum/2
  Ki/1 -> Integrator/1
  "  "/1 -> Ki/1, Kp/1
  Sum/1 -> " "/1

== system subsystem_118_bus/Linear 118 Bus ROM/Subsystem3/area3/ibr/gfm/DQ//dq ==
  D_quantity : Inport
  Q_quantity : Inport  Port=2
  theta : Inport  Port=3
  Complex to Magnitude-Angle : ComplexToMagnitudeAngle
  Complex to Real-Imag : ComplexToRealImag
  Magnitude-Angle to Complex : MagnitudeAngleToComplex
  Real-Imag to Complex : RealImagToComplex
  Sum : Sum  Inputs=|+-
  d_quantity : Outport
  q_quantity : Outport  Port=2
  wires:
  D_quantity/1 -> Real-Imag to Complex/1
  Complex to Magnitude-Angle/2 -> Sum/1
  Complex to Magnitude-Angle/1 -> Magnitude-Angle to Complex/1
  Real-Imag to Complex/1 -> Complex to Magnitude-Angle/1
  Sum/1 -> Magnitude-Angle to Complex/2
  Q_quantity/1 -> Real-Imag to Complex/2
  Magnitude-Angle to Complex/1 -> Complex to Real-Imag/1
  Complex to Real-Imag/1 -> d_quantity/1
  Complex to Real-Imag/2 -> q_quantity/1
  theta/1 -> Sum/2

== system subsystem_118_bus/Linear 118 Bus ROM/Subsystem3/area3/ibr/gfm/Subsystem1 ==
  vbDQ : Inport
  IbDQ : Inport  Port=2
  Complex to Real-Imag : ComplexToRealImag
  Complex to Real-Imag1 : ComplexToRealImag
  Product{,1..3} (4 alike) : Product
  Sum : Sum
  Sum1 : Sum  Inputs=+-
  Pm : Outport
  Qm : Outport  Port=2
  wires:
  Product/1 -> Sum/1
  Product1/1 -> Sum/2
  Sum/1 -> Pm/1
  Sum1/1 -> Qm/1
  Product3/1 -> Sum1/2
  Product2/1 -> Sum1/1
  [vbQ] -> Product2/1
  [IbD] -> Product2/2
  [vbD] -> Product3/1
  [IbQ] -> Product3/2
  [vbD] -> Product/1
  [IbD] -> Product/2
  [IbQ] -> Product1/2
  [vbQ] -> Product1/1
  vbDQ/1 -> Complex to Real-Imag/1
  Complex to Real-Imag/1 -> [vbD]
  Complex to Real-Imag/2 -> [vbQ]
  IbDQ/1 -> Complex to Real-Imag1/1
  Complex to Real-Imag1/1 -> [IbD]
  Complex to Real-Imag1/2 -> [IbQ]

== system subsystem_118_bus/Linear 118 Bus ROM/Subsystem3/area3/ibr/gfm/dq//DQ ==
  d-quantity : Inport
  q-quantity : Inport  Port=2
  theta : Inport  Port=3
  Complex to Magnitude-Angle : ComplexToMagnitudeAngle
  Complex to Real-Imag : ComplexToRealImag
  Magnitude-Angle to Complex : MagnitudeAngleToComplex
  Real-Imag to Complex : RealImagToComplex
  Sum : Sum  Inputs=|++
  D-quantity : Outport
  Q-quantity : Outport  Port=2
  wires:
  d-quantity/1 -> Real-Imag to Complex/1
  Complex to Magnitude-Angle/2 -> Sum/1
  Complex to Magnitude-Angle/1 -> Magnitude-Angle to Complex/1
  Real-Imag to Complex/1 -> Complex to Magnitude-Angle/1
  Sum/1 -> Magnitude-Angle to Complex/2
  q-quantity/1 -> Real-Imag to Complex/2
  Magnitude-Angle to Complex/1 -> Complex to Real-Imag/1
  Complex to Real-Imag/1 -> D-quantity/1
  Complex to Real-Imag/2 -> Q-quantity/1
  theta/1 -> Sum/2

== system subsystem_118_bus/Linear 118 Bus ROM/Subsystem3/area3/ibr/gfm/filter capacitor dynamics ==
  i_cf_d : Inport
  w : Inport  Port=2
  i_cf_q : Inport  Port=3
  1/C_gfm : Gain  Gain=1./Subsystem.gfm.c
  "1/C_gfm " : Gain  Gain=1./Subsystem.gfm.c
  Display : Display
  Integrator : Integrator  InitialCondition=Subsystem.gfm.v_d  ContinuousStateAttributes='gfm_vd'
  Integrator1 : Integrator  InitialCondition=Subsystem.gfm.v_q  ContinuousStateAttributes='gfm_vq'
  Product : Product
  Product1 : Product
  Sum2 : Sum  Inputs=+-
  Sum3 : Sum
  v_gfl_d : Outport
  v_gfl_q : Outport  Port=2
  wires:
  w/1 -> [ws]
  [ws] -> Product/1
  Integrator/1 -> Product1/1, v_gfl_d/1
  Integrator1/1 -> Product/2, v_gfl_q/1
  [ws] -> Product1/2
  Sum3/1 -> Display/1, Integrator/1
  Sum2/1 -> Integrator1/1
  1/C_gfm/1 -> Sum3/2
  Product/1 -> Sum3/1
  "1/C_gfm "/1 -> Sum2/1
  Product1/1 -> Sum2/2
  i_cf_d/1 -> 1/C_gfm/1
  i_cf_q/1 -> "1/C_gfm "/1

== system subsystem_118_bus/Linear 118 Bus ROM/Subsystem3/area3/ibr/gfm/p measurement delay ==
  in : Inport
  Integrator1 : Integrator  InitialCondition=Subsystem.gfm.p_ref  ContinuousStateAttributes='gfm_p_m'
  Sum2 : Sum  Inputs=-+
  p_meas_bw : Gain  Gain=Subsystem.gfm.p_meas_w
  out : Outport
  wires:
  in/1 -> Sum2/2
  Sum2/1 -> p_meas_bw/1
  Integrator1/1 -> Sum2/1, out/1
  p_meas_bw/1 -> Integrator1/1

== system subsystem_118_bus/Linear 118 Bus ROM/Subsystem3/area3/ibr/gfm/q measurement delay ==
  in : Inport
  Integrator1 : Integrator  InitialCondition=Subsystem.gfm.q_ref  ContinuousStateAttributes='gfm_q_m'
  Sum2 : Sum  Inputs=-+
  p_meas_bw : Gain  Gain=Subsystem.gfm.p_meas_w
  out : Outport
  wires:
  p_meas_bw/1 -> Integrator1/1
  Integrator1/1 -> out/1, Sum2/1
  Sum2/1 -> p_meas_bw/1
  in/1 -> Sum2/2

== system subsystem_118_bus/Linear 118 Bus ROM/Subsystem3/area3/ibr/gfm/simplified current loop d-axis ==
  " " : Inport
  Display : Display
  Gain : Gain  Gain=Subsystem.gfm.i_loop_w
  Integrator1 : Integrator  InitialCondition=Subsystem.gfm.i_d  ContinuousStateAttributes='gfm_id_ctrl'
  Sum2 : Sum  Inputs=-+
  "  " : Outport
  wires:
  Gain/1 -> Display/1, Integrator1/1
  Integrator1/1 -> "  "/1, Sum2/1
  Sum2/1 -> Gain/1
  " "/1 -> Sum2/2

== system subsystem_118_bus/Linear 118 Bus ROM/Subsystem3/area3/ibr/gfm/simplified current loop q-axis ==
  " " : Inport
  Gain : Gain  Gain=Subsystem.gfm.i_loop_w
  Integrator1 : Integrator  InitialCondition=Subsystem.gfm.i_q  ContinuousStateAttributes='gfm_iq_ctrl'
  Sum2 : Sum  Inputs=-+
  "  " : Outport
  wires:
  " "/1 -> Sum2/2
  Sum2/1 -> Gain/1
  Integrator1/1 -> Sum2/1, "  "/1
  Gain/1 -> Integrator1/1

== system subsystem_118_bus/Linear 118 Bus ROM/Subsystem3/area3/ibr/gfm/v measurement delay ==
  in : Inport
  Integrator1 : Integrator  InitialCondition=Subsystem.gfm.v_ref  ContinuousStateAttributes='gfm_v_m'
  Sum2 : Sum  Inputs=-+
  v_meas_bw : Gain  Gain=Subsystem.gfm.q_meas_w
  out : Outport
  wires:
  v_meas_bw/1 -> Integrator1/1
  Integrator1/1 -> out/1, Sum2/1
  Sum2/1 -> v_meas_bw/1
  in/1 -> Sum2/2

== system subsystem_118_bus/Linear 118 Bus ROM/Subsystem3/area3/ibr/gfm/vd_loop_pi ==
  "  " : Inport
  Integrator : Integrator  ContinuousStateAttributes='gfm_vd_ctrl'
  Ki : Gain  Gain=Subsystem.gfm_gains.vd_ki
  Kp : Gain  Gain=Subsystem.gfm_gains.vd_kp
  Sum : Sum  Inputs=|++
  " " : Outport
  wires:
  Kp/1 -> Sum/1
  Integrator/1 -> Sum/2
  Ki/1 -> Integrator/1
  "  "/1 -> Ki/1, Kp/1
  Sum/1 -> " "/1

== system subsystem_118_bus/Linear 118 Bus ROM/Subsystem3/area3/ibr/gfm/vq_loop_pi ==
  "  " : Inport
  Integrator : Integrator  ContinuousStateAttributes='gfm_vq_ctrl'
  Ki : Gain  Gain=Subsystem.gfm_gains.vq_ki
  Kp : Gain  Gain=Subsystem.gfm_gains.vq_kp
  Sum : Sum  Inputs=|++
  " " : Outport
  wires:
  Sum/1 -> " "/1
  "  "/1 -> Kp/1, Ki/1
  Ki/1 -> Integrator/1
  Integrator/1 -> Sum/2
  Kp/1 -> Sum/1

== system subsystem_118_bus/Linear 118 Bus ROM/Subsystem3/area3/non_ibr/floating buses/line charging dynamics ==
  note: I am multiplying here by negative
  note: I am multiplying here by negative
  i_float_D : Inport
  i_float_Q : Inport  Port=2
  " " : Integrator  InitialCondition=Subsystem.float.v_D  ContinuousStateAttributes='floatvD'
  1/C_float : Gain  Gain=-1./Subsystem.float.c
  "1/C_float " : Gain  Gain=-1./Subsystem.float.c
  Constant : Constant  Value=w
  Integrator1 : Integrator  InitialCondition=Subsystem.float.v_Q  ContinuousStateAttributes='floatvQ'
  Product : Product
  Product1 : Product
  Sum2 : Sum  Inputs=+-
  Sum3 : Sum
  v_float_D : Outport
  v_float_Q : Outport  Port=2
  wires:
  " "/1 -> Product1/1, v_float_D/1
  Integrator1/1 -> v_float_Q/1, Product/2
  [ws] -> Product1/2
  Sum3/1 -> " "/1
  Sum2/1 -> Integrator1/1
  1/C_float/1 -> Sum3/2
  Product/1 -> Sum3/1
  "1/C_float "/1 -> Sum2/1
  Product1/1 -> Sum2/2
  i_float_D/1 -> 1/C_float/1
  i_float_Q/1 -> "1/C_float "/1
  [ws] -> Product/1
  Constant/1 -> [ws]

== system subsystem_118_bus/Linear 118 Bus ROM/Subsystem3/area3/non_ibr/load buses/Subsystem ==
  p : Inport
  q : Inport  Port=2
  vD : Inport  Port=3
  vQ : Inport  Port=4
  Complex to Real-Imag : ComplexToRealImag
  Conj : Math  Operator=conj
  Divide : Product  Inputs=*/
  Real-Imag to Complex : RealImagToComplex
  Real-Imag to Complex1 : RealImagToComplex
  i_inj_load_d : Outport
  i_inj_load_q : Outport  Port=2
  wires:
  q/1 -> Real-Imag to Complex/2
  Real-Imag to Complex1/1 -> Divide/2
  Divide/1 -> Conj/1
  Complex to Real-Imag/2 -> i_inj_load_q/1
  Real-Imag to Complex/1 -> Divide/1
  vQ/1 -> Real-Imag to Complex1/2
  vD/1 -> Real-Imag to Complex1/1
  Complex to Real-Imag/1 -> i_inj_load_d/1
  p/1 -> Real-Imag to Complex/1
  Conj/1 -> Complex to Real-Imag/1

== system subsystem_118_bus/Linear 118 Bus ROM/Subsystem3/area3/non_ibr/load buses/line charging dynamics ==
  i_load_c_D : Inport
  i_load_c_Q : Inport  Port=2
  " " : Integrator  InitialCondition=Subsystem.load1.v_D  ContinuousStateAttributes='loadvD'
  1/C_load : Gain  Gain=1./Subsystem.load1.c
  "1/C_load " : Gain  Gain=1./Subsystem.load1.c
  Constant : Constant  Value=w
  Integrator1 : Integrator  InitialCondition=Subsystem.load1.v_Q  ContinuousStateAttributes='loadvQ'
  Product : Product
  Product1 : Product
  Sum2 : Sum  Inputs=+-
  Sum3 : Sum
  v_load_D : Outport
  v_load_Q : Outport  Port=2
  wires:
  [ws] -> Product/1
  " "/1 -> Product1/1, v_load_D/1
  Integrator1/1 -> v_load_Q/1, Product/2
  [ws] -> Product1/2
  Sum3/1 -> " "/1
  Sum2/1 -> Integrator1/1
  1/C_load/1 -> Sum3/2
  Product/1 -> Sum3/1
  "1/C_load "/1 -> Sum2/1
  Product1/1 -> Sum2/2
  i_load_c_D/1 -> 1/C_load/1
  i_load_c_Q/1 -> "1/C_load "/1
  Constant/1 -> [ws]
